simulink model "PWM_Single_Phase"  (R2021a)
settings: Solver=VariableStepDiscrete  StartTime=0.0  StopTime=0.4  MaxStep=0.001  RelTol=1e-3
libraries: simulink x1, spspowerguiLib x1
settings Model: Creator=SA  LastModifiedBy=SA

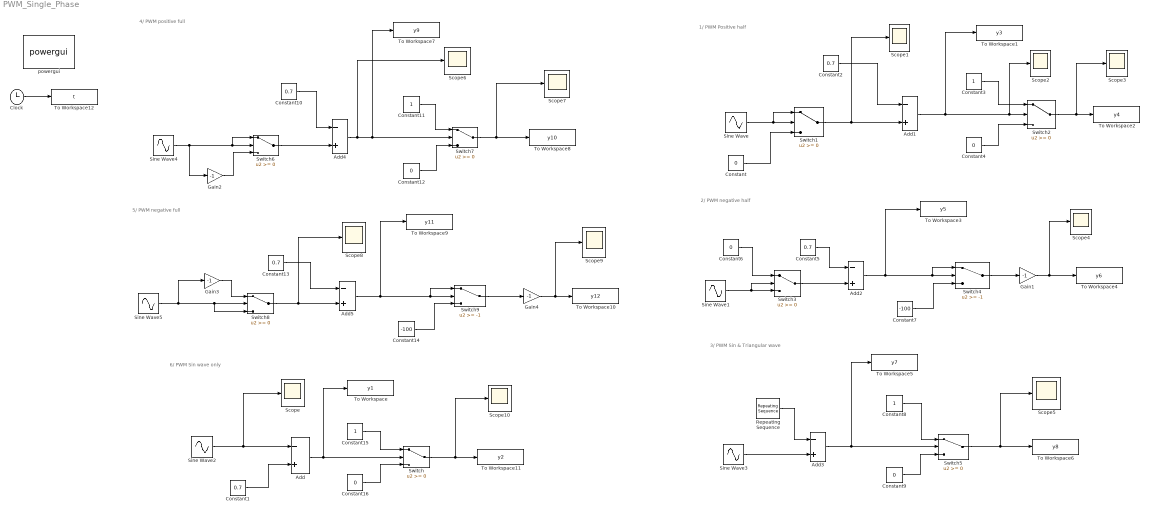
== system PWM_Single_Phase ==
  note: 6/ PWM Sin wave only
  note: 5/ PWM negative full
  note: 4/ PWM positive full
  note: 3/ PWM Sin & Triangular wave
  note: 2/ PWM negative half
  note: 1/ PWM Positive half
  Add{,1..5} (6 alike) : Sum  Inputs=-+
  Clock : Clock
  Constant{,4,6,9,12,16} (6 alike) : Constant  Value=0
  Constant{1..2,5,10,13} (5 alike) : Constant  Value=0.7
  Constant{3,8,11,15} (4 alike) : Constant
  Constant14 : Constant  Value=-100
  Constant7 : Constant  Value=-100
  Gain{1..4} (4 alike) : Gain  Gain=-1
  Repeating Sequence : simulink/Sources/Repeating Sequence  rep_seq_t=[0 0.1]  rep_seq_y=[0 0.9]
  Scope{,1..10} (11 alike) : Scope
  Sine Wave{,1..5} (6 alike) : Sin  Frequency=60  SampleTime=0
  Switch{,1..3,5..8} (8 alike) : Switch
  Switch4 : Switch  Threshold=-1
  Switch9 : Switch  Threshold=-1
  To Workspace : ToWorkspace  VariableName=y1  SaveFormat=Timeseries  SampleTime=-1
  To Workspace1 : ToWorkspace  VariableName=y3  SaveFormat=Timeseries  SampleTime=-1
  To Workspace10 : ToWorkspace  VariableName=y12  SaveFormat=Timeseries  SampleTime=-1
  To Workspace11 : ToWorkspace  VariableName=y2  SaveFormat=Timeseries  SampleTime=-1
  To Workspace12 : ToWorkspace  VariableName=t  SaveFormat=Timeseries  SampleTime=-1
  To Workspace2 : ToWorkspace  VariableName=y4  SaveFormat=Timeseries  SampleTime=-1
  To Workspace3 : ToWorkspace  VariableName=y5  SaveFormat=Timeseries  SampleTime=-1
  To Workspace4 : ToWorkspace  VariableName=y6  SaveFormat=Timeseries  SampleTime=-1
  To Workspace5 : ToWorkspace  VariableName=y7  SaveFormat=Timeseries  SampleTime=-1
  To Workspace6 : ToWorkspace  VariableName=y8  SaveFormat=Timeseries  SampleTime=-1
  To Workspace7 : ToWorkspace  VariableName=y9  SaveFormat=Timeseries  SampleTime=-1
  To Workspace8 : ToWorkspace  VariableName=y10  SaveFormat=Timeseries  SampleTime=-1
  To Workspace9 : ToWorkspace  VariableName=y11  SaveFormat=Timeseries  SampleTime=-1
  powergui : spspowerguiLib/powergui  Priority=1  SimulationMode=Discrete  SampleTime=5e-05  frequency=60  Iterations=50  frequencyindice=60  Pbase=100e6  ErrMax=1e-4  UnitsV=kV  UnitsW=MW  buscounter=0  FunctionMessages=off  echomessages=off  EnableUseOfTLC=off  CurrentSourceSwitches=off  DisableSnubberDevices=off  DisableRonSwitches=off  DisableVfSwitches=off  DisplayEquations=off  AutomaticDiscreteSolvers=off  SolverType=Tustin/Backward Euler (TBE)  Interpol=off  ExternalGateDelay=off  methode=off  Ts=100  x0status=blocks  SPID=on  SwTol=0  HookPort=off  NonlinearTolerance=1e-4  nMaxIteration=100  ContinueOnMaxIteration=off  RestoreLinks=warning  ResistiveCurrentMeasurement=off  Frange=[0:2:500]  Ylog=off  Xlog=on  ShowGrid=off  save=off  variable=ZData  structure=0  ZoomFFT=off  StartTime=0.0  cycles=1  DisplayStyle=1  fundamental=60  FreqAxis=off  MaxFrequency=1000  frequencyindicesteady=1  RmsSteady=1  display=off
  wires:
  Constant/1 -> Switch1/3
  Sine Wave/1 -> Switch1/1, Switch1/2
  Switch1/1 -> Add1/2, Scope1/1
  Constant2/1 -> Add1/1
  Add1/1 -> To Workspace1/1, Scope2/1, Switch2/2
  Constant4/1 -> Switch2/3
  Constant3/1 -> Switch2/1
  Switch2/1 -> Scope3/1, To Workspace2/1
  Sine Wave1/1 -> Switch3/2, Switch3/3
  Constant6/1 -> Switch3/1
  Constant5/1 -> Add2/1
  Switch3/1 -> Add2/2
  Constant7/1 -> Switch4/3
  Add2/1 -> To Workspace3/1, Switch4/1, Switch4/2
  Switch4/1 -> Gain1/1
  Gain1/1 -> Scope4/1, To Workspace4/1
  Sine Wave3/1 -> Add3/2
  Repeating Sequence/1 -> Add3/1
  Add3/1 -> To Workspace5/1, Switch5/2
  Constant8/1 -> Switch5/1
  Constant9/1 -> Switch5/3
  Switch5/1 -> Scope5/1, To Workspace6/1
  Switch6/1 -> Add4/2
  Constant10/1 -> Add4/1
  Sine Wave4/1 -> Gain2/1, Switch6/1, Switch6/2
  Gain2/1 -> Switch6/3
  Add4/1 -> Scope6/1, To Workspace7/1, Switch7/2
  Constant11/1 -> Switch7/1
  Constant12/1 -> Switch7/3
  Switch7/1 -> Scope7/1, To Workspace8/1
  Sine Wave5/1 -> Gain3/1, Switch8/3, Switch8/2
  Switch8/1 -> Scope8/1, Add5/2
  Constant13/1 -> Add5/1
  Gain3/1 -> Switch8/1
  Add5/1 -> To Workspace9/1, Switch9/1, Switch9/2
  Constant14/1 -> Switch9/3
  Switch9/1 -> Gain4/1
  Gain4/1 -> Scope9/1, To Workspace10/1
  Sine Wave2/1 -> Scope/1, Add/1
  Constant1/1 -> Add/2
  Add/1 -> To Workspace/1, Switch/2
  Constant15/1 -> Switch/1
  Constant16/1 -> Switch/3
  Switch/1 -> Scope10/1, To Workspace11/1
  Clock/1 -> To Workspace12/1
